simulink model "MPU6050_acq_sf_n_Working_Model"  (R2023b)
settings: Solver=FixedStepAuto  StartTime=0.0  StopTime=inf  RelTol=1e-3  EnableMultiTasking=on
libraries: arduinolib x2
settings Model: ExtModeTrigDuration=2  Creator=Marc  LastModifiedBy=jerss
settings SolverCC: AlgebraicLoopSolver=TrustRegion
settings DataIOCC: ReturnWorkspaceOutputs=off
settings OptimizationCC: EnhancedBackFolding=on  PassReuseOutputArgsAs=Individual arguments  MaxStackSize=64  OptimizeBlockOrder=speed  DifferentSizesBufferReuse=on  OptimizationCustomize=off  EfficientTunableParamExpr=on
settings DebuggingCC: ParameterTunabilityLossMsg=error  UnconnectedInputMsg=warning  UnconnectedOutputMsg=warning  UnconnectedLineMsg=warning  ArithmeticOperatorsInVariantConditions=warning
settings HardwareCC: ProdBitPerInt=16  ProdBitPerPointer=16  ProdBitPerSizeT=16  ProdBitPerPtrDiffT=16  ProdLargestAtomicFloat=None  ProdWordSize=8  ProdHWDeviceType=Atmel->AVR  UseEmbeddedCoderFeatures=off
settings ModelReferenceCC: EnableRefExpFcnMdlSchedulingChecks=on
settings SFSimCC: SimUseLocalCustomCode=off  MATLABDynamicMemAlloc=off  CustomCodeUndefinedFunction=UseInterfaceOnly
settings RTWCC: Description=Embedded Coder  SystemTargetFile=ert.tlc  HardwareBoard=Arduino Uno  TemplateMakefile=ert_default_tmf  GenerateReport=on  RTWUseLocalCustomCode=off  Toolchain=Arduino AVR  BuildConfiguration=Faster Runs  IncludeHyperlinkInReport=on  LaunchReport=on  GenerateTraceInfo=on  GenerateTraceReport=on  GenerateTraceReportSl=on  GenerateTraceReportSf=on  GenerateTraceReportEml=on
settings CodeAppCC: ForceParamTrailComments=on  IgnoreCustomStorageClasses=off  OperatorAnnotations=on  SimulinkDataObjDesc=on  SFDataObjDesc=on  InsertBlockDesc=on
settings ERTTargetCC: SupportContinuousTime=on  SupportNonInlinedSFcns=on  SupportVariableSizeSignals=on  ExtModeTransport=3  ExtModeStaticAlloc=on  ExtModeAutomaticAllocSize=off  ExtModeStaticAllocSize=250  ExtModeMexFile=ext_xcp  ExtModeIntrfLevel=Level2 - Open

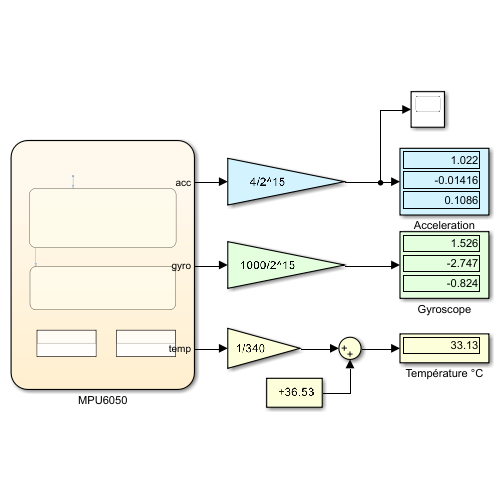
[thumbnail: Simulink's stored preview of the top-level diagram]
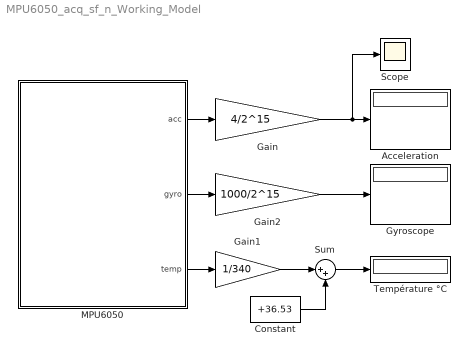
== system MPU6050_acq_sf_n_Working_Model ==
  Acceleration : Display
  Constant : Constant  Value=+36.53  OutDataTypeStr=single
  Gain : Gain  Gain=4/2^15  OutDataTypeStr=single
  Gain1 : Gain  Gain=1/340  OutDataTypeStr=single
  Gain2 : Gain  Gain=1000/2^15  OutDataTypeStr=single
  Gyroscope : Display
  MPU6050 : Stateflow chart  TreatAsAtomicUnit=on
  Scope : Scope
  Sum : Sum  Inputs=|++
  Température °C : Display
  wires:
  Sum/1 -> Température °C/1
  Constant/1 -> Sum/2
  Gain1/1 -> Sum/1
  Gain2/1 -> Gyroscope/1
  MPU6050/3(temp) -> Gain1/1
  MPU6050/2(gyro) -> Gain2/1
  Gain/1 -> Scope/1, Acceleration/1
  MPU6050/1(acc) -> Gain/1

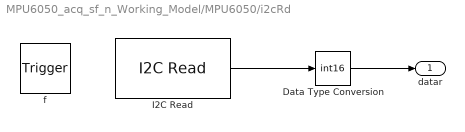
== system MPU6050_acq_sf_n_Working_Model/MPU6050/i2cRd ==
  f : TriggerPort  TriggerType=function-call  VariantControl=Variant  SampleTime=inf
      settings: CopyFcn=Stateflow.SLINSF.SimulinkMan.removeBlockPreDeleteFcn  PreDeleteFcn=Stateflow.SLINSF.SimulinkMan.unsafePredeleteFcn
  Data Type Conversion : DataTypeConversion  OutDataTypeStr=int16  SaturateOnIntegerOverflow=off  RndMeth=Floor
  I2C Read : arduinolib/I2C Read  I2CModule=0  Mode=Master  SlaveAddress=hex2dec( '68' )  SlaveByteOrder=BigEndian  Direction=Receiver  RegisterAddressMode=on  RegisterAddress=hex2dec( '3b' )  SlaveDataType=uint16  DataLength=7  NoAck=off  RepeatedStart=off  OutputStatus=off  blockPlatform=arduino  SampleTime=-1
  datar : Outport  OutDataTypeStr=int16  Unit=1  PortDimensions=7  VectorParamsAs1DForOutWhenUnconnected=off
  wires:
  I2C Read/1 -> Data Type Conversion/1
  Data Type Conversion/1 -> datar/1

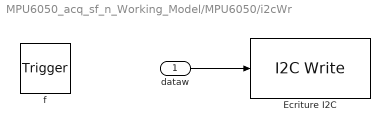
== system MPU6050_acq_sf_n_Working_Model/MPU6050/i2cWr ==
  dataw : Inport  OutDataTypeStr=uint16  Unit=1  PortDimensions=1
  f : TriggerPort  TriggerType=function-call  VariantControl=Variant  SampleTime=-1
      settings: CopyFcn=Stateflow.SLINSF.SimulinkMan.removeBlockPreDeleteFcn  PreDeleteFcn=Stateflow.SLINSF.SimulinkMan.unsafePredeleteFcn
  Ecriture I2C : arduinolib/I2C Write  Priority=1  I2CModule=0  Mode=Master  SlaveAddress=hex2dec( '68' )  SlaveByteOrder=BigEndian  Direction=Transmitter  RegisterAddressMode=off  RegisterAddress=hex2dec( '6B' )  SlaveDataType=uint16  DataLength=1  NoAck=off  RepeatedStart=off  OutputStatus=off  blockPlatform=arduino
  wires:
  dataw/1 -> Ecriture I2C/1

== stateflow chart MPU6050_acq_sf_n_Working_Model/MPU6050 ==
  state initialisation
    en:
    i2cWr(uint16(hex2dec( '6B00' )));%Power on
    i2cWr(uint16(hex2dec( '1B10' )));%gyro 0x10=1000°/s
    i2cWr(uint16(hex2dec( '1C08' )));%acce 0x08= 4G
    i2cWr(uint16(hex2dec( '1A06' )));%filtrage+actu 0x06= 19ms
    i2cWr(uint16(hex2dec( '3710' )));%INT_PIN_CFG
    i2cWr(uint16(hex2dec( '3800' )));%Interrupt Enable 0 désactivé
  state Lecture_acceleration3_axes
    during:
    val=i2cRd;
    acc=val(1:3);
    gyro=val(5:7);
    temp=val(4:4);
  state i2cWr(dataw) [function]
  state datar = i2cRd [function]
  (default) -> initialisation
  initialisation -> Lecture_acceleration3_axes
  data: dataw function_input uint16 size=1; datar function_output int16 size=7; acc output int16 size=3; gyro output int16 size=3; val local int16 size=7; temp output int16 size=1
